simulink model "control_system_obs"  (R2020a)
settings: Solver=VariableStepAuto  StartTime=0.0  StopTime=1000  RelTol=1e-3
InitFcn:
  | LAB2
values from neighbouring files (symbols this model uses):
  A = [-0.342 0 0.0318; 0 -0.0716 0.0318; 0.0204 0.0204 -0.0423]    [LAB2.m]
  B = [0.159 0; 0 0.159; 0 0]    [LAB2.m]
  C = [1 0 0; 0 1 0]    [LAB2.m]
  K = K_(:,1:3)    [LAB2.m]
  L = L'    [LAB2.m]
  N = K_(:,4:end)    [LAB2.m]
settings Model: Creator=paulogil  LastModifiedBy=joaom
settings OptimizationCC: LifeSpan=inf
settings DebuggingCC: SFExecutionAtInitializationDiag=none  ArithmeticOperatorsInVariantConditions=warning
settings SFSimCC: CustomCodeUndefinedFunction=UseInterfaceOnly
settings CodeAppCC: StateflowObjectComments=on

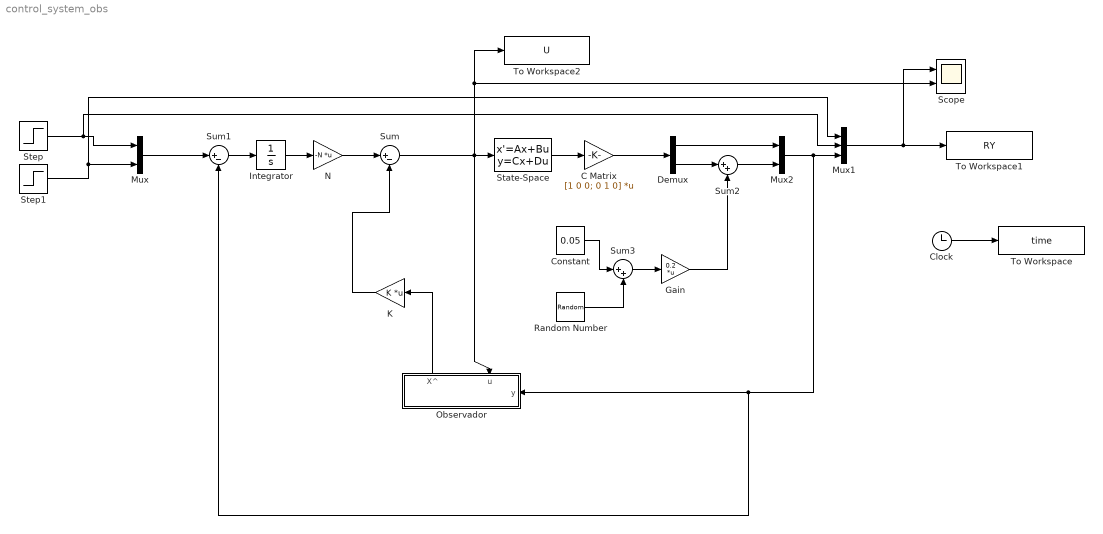
== system control_system_obs ==
  C Matrix : Gain  Gain=[1 0 0; 0 1 0]  Multiplication=Matrix(K*u)
  Clock : Clock
  Constant : Constant  Value=0.05
  Demux : Demux  Outputs=2
  Gain : Gain  Gain=0.2  Multiplication=Matrix(K*u)
  Integrator : Integrator
  K : Gain  Gain=K  Multiplication=Matrix(K*u)
  Mux : Mux  Inputs=2
  Mux1 : Mux  Inputs=3
  Mux2 : Mux  Inputs=2
  N : Gain  Gain=-N  Multiplication=Matrix(K*u)
  Observador : Subsystem
      settings: PortSchema="{\"entries\":[{\"content\":{\"sides\":[{\"content\":{\"connectorIds\":[]},\"type\":\"ConnectorPlacement.EquallySpacedRectSide\",\"uuid\":\"d5cd1a68-c78a-445d-a1e2-5900bce970fa\"},{\"content\":{\"connectorIds\":[\"In2\"],\"side\":\"RIGHT\"},\"type\":\"ConnectorPlacement.EquallySpacedRectSide\",\"uuid\":\"a187cc34-62a7-406f-881a-29c4813bd4e9\"},{\"content\":{\"connectorIds\":[\"Out1\",\"In1\"],\"side\":\"TOP\"},\"type\":\"ConnectorPlacement.EquallySpacedRectSide\",\"uuid\":\"6a3e2322-0d7f-4c39-b811-2d0822fdda52\"}]},\"type\":\"ConnectorPlacement.EquallySpacedConnector\",\"uuid\":\"1f0ac90e-7bdc-4fad-ad98-033ba63f6bbe\"}],\"packageUris\":[\"http://schema.mathworks.com/mf0/Connector/19700101\"],\"version\":\"1.0\"}"
  Random Number : RandomNumber  Variance=0.001  SampleTime=0.1
  Scope : Scope  NumInputPorts=2
  State-Space : StateSpace  A=A  B=B  C=eye(3)  D=zeros(3,2)  InitialCondition=0
  Step : Step  Time=0  After=0.7  SampleTime=0
  Step1 : Step  After=.4  SampleTime=0
  Sum : Sum  Inputs=|+-
  Sum1 : Sum  Inputs=|+-
  Sum2 : Sum  Inputs=|++
  Sum3 : Sum  Inputs=|++
  To Workspace : ToWorkspace  VariableName=time  SaveFormat=Timeseries  SampleTime=-1
  To Workspace1 : ToWorkspace  VariableName=RY  SaveFormat=Timeseries  SampleTime=-1
  To Workspace2 : ToWorkspace  VariableName=U  SaveFormat=Timeseries  SampleTime=-1
  wires:
  State-Space/1 -> C Matrix/1
  K/1 -> Sum/2
  N/1 -> Sum/1
  Mux1/1 -> To Workspace1/1, Scope/1
  Clock/1 -> To Workspace/1
  Integrator/1 -> N/1
  Sum1/1 -> Integrator/1
  Step/1 -> Mux1/2, Mux/1
  Step1/1 -> Mux1/1, Mux/2
  Mux/1 -> Sum1/1
  Observador/1(X^) -> K/1
  Sum/1 -> Scope/2, To Workspace2/1, Observador/1(u), State-Space/1
  Gain/1 -> Sum2/2
  Sum3/1 -> Gain/1
  Constant/1 -> Sum3/1
  Random Number/1 -> Sum3/2
  C Matrix/1 -> Demux/1
  Demux/1 -> Mux2/1
  Demux/2 -> Sum2/1
  Sum2/1 -> Mux2/2
  Mux2/1 -> Sum1/2, Observador/2(y), Mux1/3

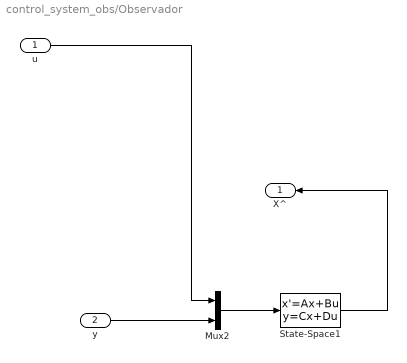
== system control_system_obs/Observador ==
  u : Inport
  y : Inport  Port=2
  Mux2 : Mux  Inputs=2
  State-Space1 : StateSpace  A=A-L*C  B=[B L]  C=eye(3)  D=zeros(3,4)  InitialCondition=[0.05 0.02 0.01]'
  X^ : Outport
  wires:
  u/1 -> Mux2/1
  Mux2/1 -> State-Space1/1
  y/1 -> Mux2/2
  State-Space1/1 -> X^/1
